simulink model "Treadmill_SPT"  (R2017b)
settings: Solver=FixedStepDiscrete  StartTime=0.0  StopTime=inf  FixedStep=0.001  RelTol=1e-3  EnableMultiTasking=on
undefined symbols (not defined in the file or in its folder): DiscIntNeverNeededParam
libraries: speedgoatlib_IO106 x2, slrtlib x1
settings Model: sg_rtwmakecfg_data=_sglibc_  Creator=Katie  LastModifiedBy=Vicon-OEM
settings SolverCC: ConcurrentTasks=on  AutoInsertRateTranBlk=on
settings DataIOCC: SaveFormat=StructureWithTime  SaveOutput=off  SaveTime=off
settings OptimizationCC: BlockReduction=off  OptimizeBlockIOStorage=off  BufferReuse=off  GlobalBufferReuse=off  ExpressionFolding=off  LocalBlockOutputs=off
settings HardwareCC: ProdBitPerPointer=32  ProdBitPerSizeT=32  ProdBitPerPtrDiffT=32  ProdLargestAtomicFloat=None  ProdWordSize=32  ProdLongLongMode=on  ProdHWDeviceType=Generic->32-bit x86 compatible
settings RTWCC: SystemTargetFile=slrt.tlc  TemplateMakefile=slrt_default_tmf  Description=Simulink Real-Time  CodeExecutionProfiling=on  RTWCompilerOptimization=on
settings SimulinkRealTimeCC: SupportVariableSizeSignals=on  RL32LogTETModifier=off  xPCConcurrentTasks=on

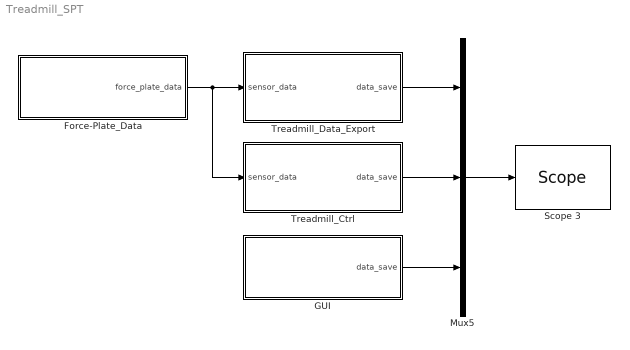
== system Treadmill_SPT ==
  Force-Plate_Data : Subsystem
  GUI : Subsystem
  Mux5 : Mux  Inputs=3
  Scope 3 : slrtlib/Displays and Logging/Scope   scopeno=101  scopetype=File  autostart=off  viewmode=Graphical redraw  formatstr='%15.6f'  grid=on  ylimits=[0,0]  nosamples=60*60*1000  noprepostsamples=0  interleave=1  triggermode=FreeRun  triggersignal=1  trigsignalfromport=off  triggerlevel=0.0  triggerslope=Either  triggerscope=1  triggersample=0  filename=pacedTM.dat  mode=Lazy  writesize=512  autorestart=off  dynamicfilemode=off  maxwritefilesize=512*1024^2
  Treadmill_Ctrl : Subsystem
  Treadmill_Data_Export : Subsystem
  wires:
  Force-Plate_Data/1(force_plate_data) -> Treadmill_Ctrl/1(sensor_data), Treadmill_Data_Export/1(sensor_data)
  Treadmill_Data_Export/1(data_save) -> Mux5/1
  Treadmill_Ctrl/1(data_save) -> Mux5/2
  Mux5/1 -> Scope 3/1
  GUI/1(data_save) -> Mux5/3

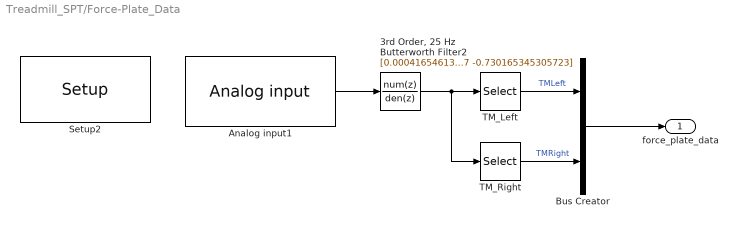
== system Treadmill_SPT/Force-Plate_Data ==
  "3rd Order, 25 Hz Butterworth Filter2" : DiscreteFilter  Numerator="[0.000416546139075769\t0.00124963841722731\t0.00124963841722731\t0.000416546139075769]"  Denominator="[1\t-2.68615739654814\t2.41965511096647\t-0.730165345305723]"
  Analog input1 : speedgoatlib_IO106/Analog input  id=1  channels=12  range=1  coupling=1  ts=dt_speedgoat  initiator=1  pciSlot=-1
      settings: SourceProductName=Simulink Real-Time: Speedgoat I/O Driver Library
  Bus Creator : BusCreator  Inputs=2
  Setup2 : speedgoatlib_IO106/Setup  group=Module setup  id=1  cal=on  initiator=Initiator  pciSlot=-1  adChannel=12  adRange=+-10V  adCoupling=Single-ended
      settings: SourceProductName=Simulink Real-Time: Speedgoat I/O Driver Library
  TM_Left : Selector  InputPortWidth=12  IndexOptions=Index vector (dialog)  Indices=1:6  OutputSizes=1
  TM_Right : Selector  InputPortWidth=12  IndexOptions=Index vector (dialog)  Indices=7:12  OutputSizes=1
  force_plate_data : Outport
  wires:
  Bus Creator/1 -> force_plate_data/1
  Analog input1/1 -> "3rd Order, 25 Hz Butterworth Filter2"/1
  "3rd Order, 25 Hz Butterworth Filter2"/1 -> TM_Right/1, TM_Left/1
  TM_Left/1 -> Bus Creator/1  "TMLeft"
  TM_Right/1 -> Bus Creator/2  "TMRight"

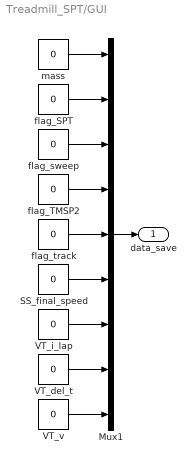
== system Treadmill_SPT/GUI ==
  Mux1 : Mux  Inputs=9
  SS_final_speed : Constant  Value=0
  VT_del_t : Constant  Value=0
  VT_i_lap : Constant  Value=0
  VT_v : Constant  Value=0
  flag_SPT : Constant  Value=0
  flag_TMSP2 : Constant  Value=0
  flag_sweep : Constant  Value=0
  flag_track : Constant  Value=0
  mass : Constant  Value=0
  data_save : Outport
  wires:
  VT_del_t/1 -> Mux1/8
  VT_v/1 -> Mux1/9
  SS_final_speed/1 -> Mux1/6
  VT_i_lap/1 -> Mux1/7
  flag_track/1 -> Mux1/5
  Mux1/1 -> data_save/1
  flag_sweep/1 -> Mux1/3
  flag_SPT/1 -> Mux1/2
  mass/1 -> Mux1/1
  flag_TMSP2/1 -> Mux1/4

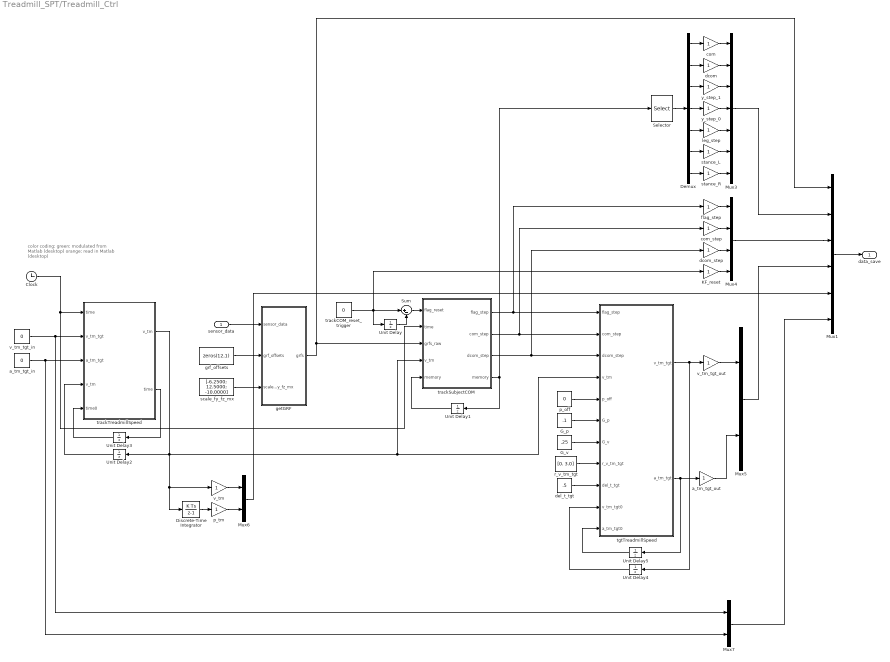
== system Treadmill_SPT/Treadmill_Ctrl ==
  note: color coding:
      | green: modulated from Matlab (desktop)
      | orange: read in Matlab (desktop)
  sensor_data : Inport
  Clock : Clock
  Demux : Demux  Outputs=7
  Discrete-Time Integrator : DiscreteIntegrator  InitialConditionSetting=State (most efficient)  SampleTime=-1  ICPrevOutput=DiscIntNeverNeededParam  ICPrevScaledInput=DiscIntNeverNeededParam
  G_p : Constant  Value=.1
  G_v : Constant  Value=.25
  KF_reset : Gain
  Mux1 : Mux  Inputs=6
  Mux3 : Mux  Inputs=7
  Mux4 : Mux
  Mux5 : Mux  Inputs=2
  Mux6 : Mux  Inputs=2
  Mux7 : Mux  Inputs=2
  Selector : Selector  InputPortWidth=82  IndexOptions=Index vector (dialog)  Indices=[2 3 13 14 11 8 9]  OutputSizes=1
  Sum : Sum  Inputs=|+-
  Unit Delay{,2..5} (5 alike) : UnitDelay  SampleTime=-1
  Unit Delay1 : UnitDelay  InitialCondition=[0 0 0 .00383 .00162 .00162 .00166 0 0 .7 0 1 .35 -.35 0 -.5 0 0 0 0 0 0 zeros(1,60)]  SampleTime=-1
  a_tm_tgt_in : Constant  Value=0
  a_tm_tgt_out : Gain
  com : Gain
  com_step : Gain
  dcom : Gain
  dcom_step : Gain
  del_t_tgt : Constant  Value=.5
  flag_step : Gain
  getGRF : Subsystem
  grf_offsets : Constant  Value=zeros(12,1)
  leg_step : Gain
  p_off : Constant  Value=0
  p_tm : Gain
  r_v_tm_tgt : Constant  Value=[0. 3.0]
  scale_fy_fz_mx : Constant  Value=[-6.2500; 12.5000; -10.0000]
  stance_L : Gain
  stance_R : Gain
  tgtTreadmillSpeed : MATLAB Function  TreatAsAtomicUnit=on
  trackCOM_reset_trigger : Constant  Value=0
  trackSubjectCOM : MATLAB Function  TreatAsAtomicUnit=on
  trackTreadmillSpeed : MATLAB Function  TreatAsAtomicUnit=on
  v_tm : Gain
  v_tm_tgt_in : Constant  Value=0
  v_tm_tgt_out : Gain
  y_step_0 : Gain
  y_step_1 : Gain
  data_save : Outport
  wires:
  com/1 -> Mux3/1
  dcom/1 -> Mux3/2
  y_step_1/1 -> Mux3/3
  sensor_data/1 -> getGRF/1(sensor_data)
  trackCOM_reset_trigger/1 -> KF_reset/1, Sum/1, Unit Delay/1
  Unit Delay/1 -> Sum/2
  Sum/1 -> trackSubjectCOM/1(flag_reset)
  trackSubjectCOM/4(memory) -> Unit Delay1/1, Selector/1
  Unit Delay1/1 -> trackSubjectCOM/5("memory ")
  trackSubjectCOM/1(flag_step) -> flag_step/1, tgtTreadmillSpeed/1(flag_step)
  trackSubjectCOM/3(dcom_step) -> tgtTreadmillSpeed/3(dcom_step), dcom_step/1
  trackTreadmillSpeed/1(v_tm) -> tgtTreadmillSpeed/4(v_tm), trackSubjectCOM/4(v_tm), Discrete-Time Integrator/1, v_tm/1, Unit Delay2/1
  Unit Delay2/1 -> trackTreadmillSpeed/4("v_tm ")
  trackTreadmillSpeed/2(time) -> Unit Delay3/1
  Unit Delay3/1 -> trackTreadmillSpeed/5(time0)
  Clock/1 -> trackSubjectCOM/2(time), trackTreadmillSpeed/1("time ")
  v_tm_tgt_in/1 -> Mux7/1, trackTreadmillSpeed/2(v_tm_tgt)
  a_tm_tgt_in/1 -> Mux7/2, trackTreadmillSpeed/3(a_tm_tgt)
  v_tm_tgt_out/1 -> Mux5/1
  a_tm_tgt_out/1 -> Mux5/2
  tgtTreadmillSpeed/2(a_tm_tgt) -> a_tm_tgt_out/1, Unit Delay5/1
  tgtTreadmillSpeed/1(v_tm_tgt) -> v_tm_tgt_out/1, Unit Delay4/1
  Selector/1 -> Demux/1
  Demux/1 -> com/1
  Demux/2 -> dcom/1
  Demux/3 -> y_step_1/1
  com_step/1 -> Mux4/2
  trackSubjectCOM/2(com_step) -> tgtTreadmillSpeed/2(com_step), com_step/1
  dcom_step/1 -> Mux4/3
  flag_step/1 -> Mux4/1
  grf_offsets/1 -> getGRF/2(grf_offsets)
  scale_fy_fz_mx/1 -> getGRF/3(scale_fy_fz_mx)
  getGRF/1(grfs) -> Mux1/1, trackSubjectCOM/3(grfs_raw)
  Unit Delay4/1 -> tgtTreadmillSpeed/10(v_tm_tgt0)
  Unit Delay5/1 -> tgtTreadmillSpeed/11(a_tm_tgt0)
  Demux/5 -> leg_step/1
  Demux/7 -> stance_R/1
  stance_L/1 -> Mux3/6
  stance_R/1 -> Mux3/7
  Demux/6 -> stance_L/1
  leg_step/1 -> Mux3/5
  y_step_0/1 -> Mux3/4
  Demux/4 -> y_step_0/1
  Mux1/1 -> data_save/1
  Mux4/1 -> Mux1/3
  Mux3/1 -> Mux1/2
  Mux5/1 -> Mux1/4
  KF_reset/1 -> Mux4/4
  Discrete-Time Integrator/1 -> p_tm/1
  p_tm/1 -> Mux6/2
  v_tm/1 -> Mux6/1
  Mux6/1 -> Mux1/5
  Mux7/1 -> Mux1/6
  G_p/1 -> tgtTreadmillSpeed/6(G_p)
  G_v/1 -> tgtTreadmillSpeed/7(G_v)
  r_v_tm_tgt/1 -> tgtTreadmillSpeed/8(r_v_tm_tgt)
  del_t_tgt/1 -> tgtTreadmillSpeed/9(del_t_tgt)
  p_off/1 -> tgtTreadmillSpeed/5(p_off)

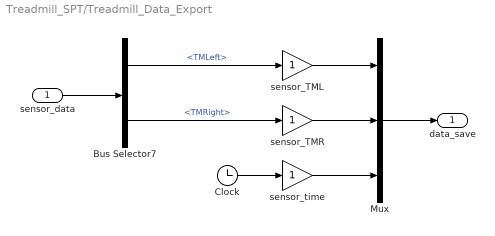
== system Treadmill_SPT/Treadmill_Data_Export ==
  sensor_data : Inport
  Bus Selector7 : BusSelector  OutputSignals=TMLeft,TMRight
  Clock : Clock
  Mux : Mux  Inputs=3
  sensor_TML : Gain
  sensor_TMR : Gain
  sensor_time : Gain
  data_save : Outport
  wires:
  Bus Selector7/1 -> sensor_TML/1  "<TMLeft>"
  Bus Selector7/2 -> sensor_TMR/1  "<TMRight>"
  sensor_data/1 -> Bus Selector7/1
  Clock/1 -> sensor_time/1
  sensor_time/1 -> Mux/3
  sensor_TMR/1 -> Mux/2
  sensor_TML/1 -> Mux/1
  Mux/1 -> data_save/1

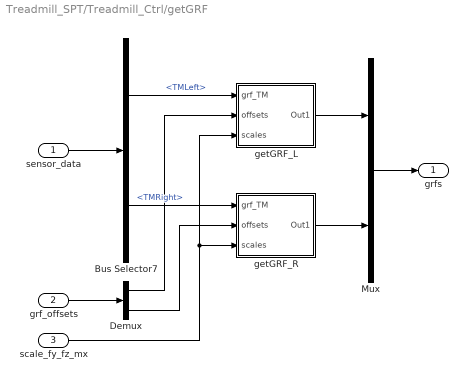
== system Treadmill_SPT/Treadmill_Ctrl/getGRF ==
  sensor_data : Inport
  grf_offsets : Inport  Port=2
  scale_fy_fz_mx : Inport  Port=3
  Bus Selector7 : BusSelector  OutputSignals=TMLeft,TMRight
  Demux : Demux  Outputs=2
  Mux : Mux  Inputs=2
  getGRF_L : Subsystem
  getGRF_R : Subsystem
  grfs : Outport
  wires:
  Bus Selector7/1 -> getGRF_L/1(grf_TM)  "<TMLeft>"
  sensor_data/1 -> Bus Selector7/1
  Mux/1 -> grfs/1
  scale_fy_fz_mx/1 -> getGRF_R/3(scales), getGRF_L/3(scales)
  Bus Selector7/2 -> getGRF_R/1(grf_TM)  "<TMRight>"
  getGRF_L/1(Out1) -> Mux/1
  getGRF_R/1(Out1) -> Mux/2
  grf_offsets/1 -> Demux/1
  Demux/1 -> getGRF_L/2(offsets)
  Demux/2 -> getGRF_R/2(offsets)

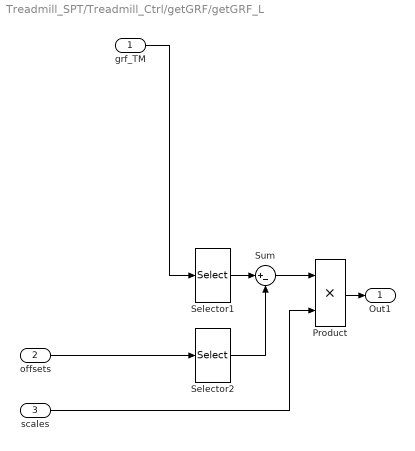
== system Treadmill_SPT/Treadmill_Ctrl/getGRF/getGRF_L ==
  grf_TM : Inport
  offsets : Inport  Port=2
  scales : Inport  Port=3
  Product : Product
  Selector1 : Selector  InputPortWidth=6  IndexOptions=Index vector (dialog)  Indices=[2 3 4]  OutputSizes=1
  Selector2 : Selector  InputPortWidth=6  IndexOptions=Index vector (dialog)  Indices=[2 3 4]  OutputSizes=1
  Sum : Sum  Inputs=|+-
  Out1 : Outport
  wires:
  Product/1 -> Out1/1
  grf_TM/1 -> Selector1/1
  scales/1 -> Product/2
  offsets/1 -> Selector2/1
  Selector1/1 -> Sum/1
  Sum/1 -> Product/1
  Selector2/1 -> Sum/2

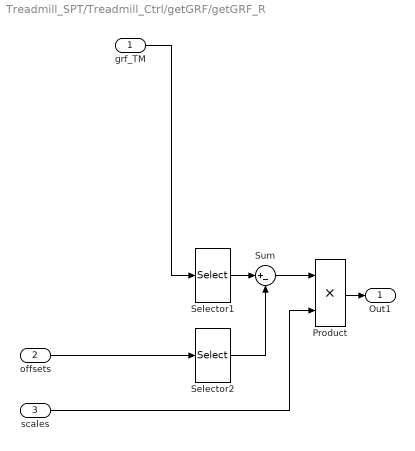
== system Treadmill_SPT/Treadmill_Ctrl/getGRF/getGRF_R ==
  grf_TM : Inport
  offsets : Inport  Port=2
  scales : Inport  Port=3
  Product : Product
  Selector1 : Selector  InputPortWidth=6  IndexOptions=Index vector (dialog)  Indices=[2 3 4]  OutputSizes=1
  Selector2 : Selector  InputPortWidth=6  IndexOptions=Index vector (dialog)  Indices=[2 3 4]  OutputSizes=1
  Sum : Sum  Inputs=|+-
  Out1 : Outport
  wires:
  Product/1 -> Out1/1
  grf_TM/1 -> Selector1/1
  scales/1 -> Product/2
  offsets/1 -> Selector2/1
  Selector1/1 -> Sum/1
  Sum/1 -> Product/1
  Selector2/1 -> Sum/2

== matlab function Treadmill_SPT/Treadmill_Ctrl/trackTreadmillSpeed ==
  data: time input; v_tm_tgt input; a_tm_tgt input; v_tm input; time0 input; v_tm output; time output
function [v_tm, time] = ...
    fcn(time, v_tm_tgt, a_tm_tgt, v_tm, time0)


del_t = time - time0;
del_v = v_tm_tgt - v_tm;
if del_v > 0
    del_v = min(del_v, a_tm_tgt*del_t);
else
    del_v = max(del_v, -a_tm_tgt*del_t);
end
v_tm = v_tm + del_v;

== matlab function Treadmill_SPT/Treadmill_Ctrl/tgtTreadmillSpeed ==
  data: flag_step input; com_step input; dcom_step input; v_tm input; p_off input; G_p input; G_v input; r_v_tm_tgt input; del_t_tgt input; v_tm_tgt output; a_tm_tgt output; v_tm_tgt0 input; a_tm_tgt0 input
function [v_tm_tgt, a_tm_tgt] = fcn(...
    flag_step, com_step, dcom_step, v_tm, ...
    p_off, G_p, G_v, r_v_tm_tgt, del_t_tgt, ...
    v_tm_tgt0, a_tm_tgt0)

[v_tm_tgt, a_tm_tgt] = speed_controller(...
    flag_step, com_step, dcom_step, v_tm, ...
    p_off, G_p, G_v, r_v_tm_tgt, del_t_tgt, ...
    v_tm_tgt0, a_tm_tgt0);

== matlab function Treadmill_SPT/Treadmill_Ctrl/trackSubjectCOM ==
  data: flag_step output; flag_reset input; time input; grfs_raw input; v_tm input; com_step output; memory input; dcom_step output; memory output
function [flag_step, com_step, dcom_step, memory] = ...
    fcn(flag_reset, time, grfs_raw, v_tm, memory)

[flag_step, com_step, dcom_step, memory] = ...
    state_estimator(flag_reset, time, grfs_raw, v_tm, memory);
